simulink model "water_hopper_biped_FCPG_split"  (Simulink 8.0)
settings: Solver=ode23t  StartTime=0.0  StopTime=6  MaxStep=1e-3  RelTol=1e-3
values from neighbouring files (symbols this model uses):
  alpha = 30    [SimParam_FCPG.m]
  Amp = 0.0249    [SimParam_FCPG.m]
  C_d = 0.703    [SimParam_FCPG.m]
  density = 1000    [SimParam_FCPG.m]
  freq = 70    [SimParam_FCPG.m]
  g = 9.81    [SimParam_FCPG.m]
  leg_length = Amp    (= 0.0249)    [SimParam_FCPG.m]
  mass = 0.05    [SimParam_FCPG.m]
  omega_0 = [60 60]'    [SimParam_FCPG.m]
  S1 = (pi*r1^2)*area    (= 0.00115422114093)    [SimParam_FCPG.m]
  S2 = (pi*r2^2)*area    (= 7.21388213081e-05)    [SimParam_FCPG.m]
  tau = 0.001    [SimParam_FCPG.m]
undefined symbols (not defined in the file or in its folder): b, Fratio, k
undefined symbols (not defined in the file): amp, RL_lag, W_coupling, y_0
libraries: mblibv1 x16, dspstat3 x1, simulink x1, dspinverses x1
settings Model: Creator=Metti  LastModifiedBy=nitisht
settings SolverCC: ZeroCrossControl=DisableAll
settings DataIOCC: SignalLoggingSaveFormat=ModelDataLogs
settings DebuggingCC: FcnCallInpInsideContextMsg=EnableAllAsWarning
settings ConfigurationSet: Description=SimMechanics 2G

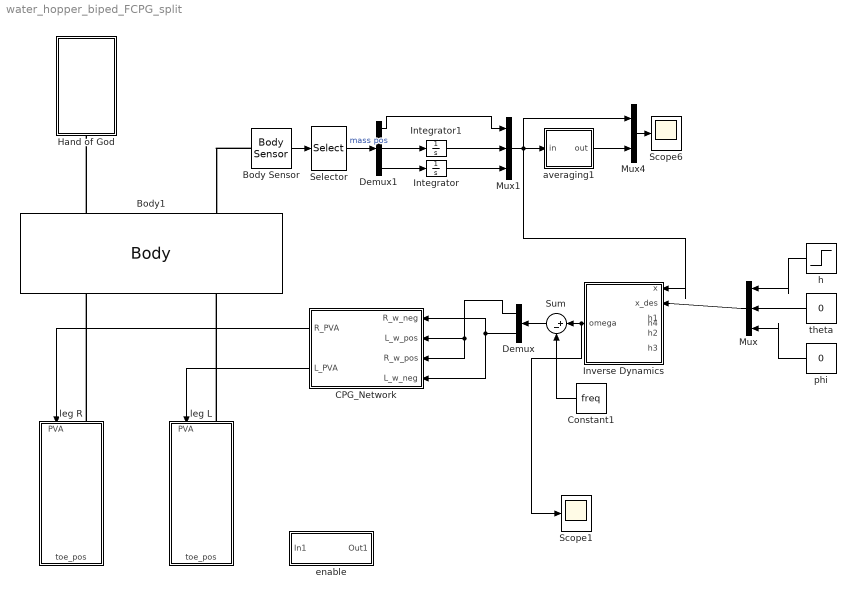
== system water_hopper_biped_FCPG_split ==
  Body Sensor : mblibv1/Sensors &  Actuators/Body Sensor  UpdateFromCAD=off  PhysicalDomain=Mechanical  PortType=blob  Muxed=on  Pose=off  Angle=on  AngleUnits=deg  ArcVelocity=on  ArcVelocityUnits=rad/s  ArcAcceleration=off  ArcAccelerationUnits=deg/s^2  CoordPosition=on  CoordPositionUnits=m  Velocity=off  VelocityUnits=m/s  Acceleration=off  AccelerationUnits=m/s^2  Quaternion=on  QuaternionDT=off  QuaternionDDT=off  QuaternionUnits=off  OutputVector=[1]  ActiveIO=on  Width=3  DialogClass=MechanicalSensorBlock  ReferenceFrame=Absolute (World)
  Body1 : mblibv1/Bodies/Body  LConnTagsString=CS1|CS2  RConnTagsString=CS3|CS4  UpdateFromCAD=off  DialogClass=MechanicalBodyBlock  Mass=mass  MassUnits=kg  InertiaUnits=kg*m^2  Inertia=eye(3)  Shape=Cylinder  ShapeDims=[1 1]  ShapeUnits=m  ShapeUse=false  Density=1  DensityUnits=kg/m^3  DensityUse=false  GraphicsMode=MACHINE_DEFAULT  BodyColorSelMode=MACHINE_DEFAULT  BodyColor=[1 0 0]  AttachedToCS=CG  CG=Left$CG$[0 0 0]$WORLD$WORLD$m$[0 0 0]$Euler X-Y-Z$deg$WORLD$false$none  WorkingFrames=Left$CS1$[0 0 0]$CG$CG$m$[0 0 0]$Euler X-Y-Z$deg$WORLD$true$none#Left$CS2$[0 0 0]$CG$CG$m$[0 0 0]$Euler X-Y-Z$deg$WORLD$true$none#Right$CS3$[0 0 0]$CG$CG$m$[0 0 0]$Euler X-Y-Z$deg$WORLD$true$none#Right$CS4$[0 0 0]$CG$CG$m$[0 0 0]$Euler X-Y-Z$deg$WORLD$true$none  CGPos=[0 0 0]  CGRot=[0 0 0]  CS0Pos=[]  CS0Rot=[]  CS1Pos=[0 0 0]  CS1Rot=[0 0 0]  CS2Pos=[0 0 0]  CS2Rot=[0 0 0]  CS3Pos=[0 0 0]  CS3Rot=[0 0 0]  CS4Pos=[0 0 0]  CS4Rot=[0 0 0]  CS5Pos=[]  CS5Rot=[]  CS6Pos=[]  CS6Rot=[]  CS7Pos=[]  CS7Rot=[]  CS8Pos=[]  CS8Rot=[]  CS9Pos=[]  CS9Rot=[]  CS10Pos=[]  CS10Rot=[]  CS11Pos=[]  CS11Rot=[]  CS12Pos=[]  CS12Rot=[]  CS13Pos=[]  CS13Rot=[]  CS14Pos=[]  CS14Rot=[]  CS15Pos=[]  CS15Rot=[]  CS16Pos=[]  CS16Rot=[]  CS17Pos=[]  CS17Rot=[]  CS18Pos=[]  CS18Rot=[]  CS19Pos=[]  CS19Rot=[]  CS20Pos=[]  CS20Rot=[]
  CPG_Network : Subsystem
  Constant1 : Constant  Value=freq
  Demux : Demux  Outputs=2
  Demux1 : Demux  Outputs=3
  Hand of God : Subsystem
  Integrator : Integrator
  Integrator1 : Integrator
  Inverse Dynamics : Subsystem
  Mux : Mux  Inputs=3
  Mux1 : Mux  Inputs=3
  Mux4 : Mux  Inputs=2
  Scope1 : Scope
      settings: TimeRange=0.00234049245184974  YMin=53.02063772134064  YMax=53.05517753304328  SaveName=omega_control
  Scope6 : Scope
      settings: YMin=0  YMax=0.0175  SaveName=ball_position
  Selector : Selector  InputPortWidth=6  IndexOptions=Index vector (dialog)  Indices=[2 4 5]  OutputSizes=1
  Sum : Sum  Inputs=|+-
  averaging1 : Subsystem  mask{T_win=2*pi/freq*2, x_init=y_0}
      mask prompts: T_win "window (s)"; x_init "Initial condition"
  enable : Subsystem
  h : Step  Time=3  Before=.01  After=.015  SampleTime=0
  leg L : Subsystem
  leg R : Subsystem
  phi : Constant  Value=0
  theta : Constant  Value=0
  wires:
  Body Sensor/1 -> Selector/1
  Mux4/1 -> Scope6/1
  CPG_Network/1(R_PVA) -> leg R/1(PVA)
  CPG_Network/2(L_PVA) -> leg L/1(PVA)
  averaging1/1(out) -> Mux4/2
  Demux/1 -> CPG_Network/3(R_w_pos), CPG_Network/2(L_w_pos)
  Demux/2 -> CPG_Network/4(L_w_neg), CPG_Network/1(R_w_neg)
  Sum/1 -> Demux/1
  Constant1/1 -> Sum/2
  Inverse Dynamics/1(omega) -> Scope1/1, Sum/1
  h/1 -> Mux/1
  theta/1 -> Mux/2
  phi/1 -> Mux/3
  Mux/1 -> Inverse Dynamics/2(x_des)
  Selector/1 -> Demux1/1  "mass pos"
  Demux1/3 -> Integrator/1
  Demux1/2 -> Integrator1/1
  Mux1/1 -> Inverse Dynamics/1(x), Mux4/1, averaging1/1(in)
  Demux1/1 -> Mux1/1
  Integrator1/1 -> Mux1/2
  Integrator/1 -> Mux1/3
  connections:
  Body Sensor/LConn1 -- Body1/LConn2
  leg R/LConn1 -- Body1/RConn1
  Body1/LConn1 -- Hand of God/LConn1
  leg L/LConn1 -- Body1/RConn2

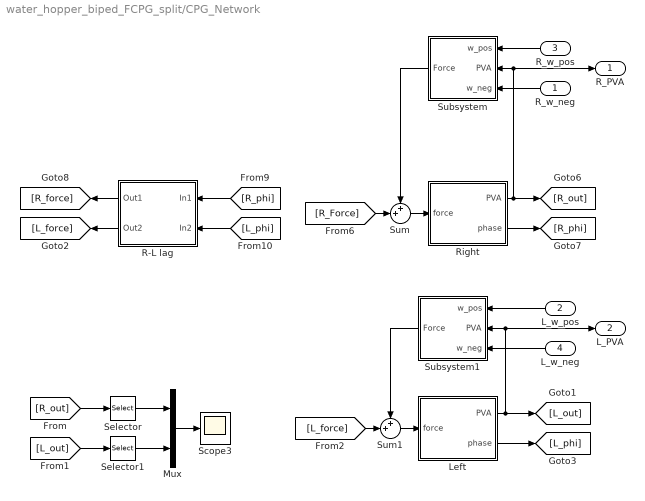
== system water_hopper_biped_FCPG_split/CPG_Network ==
  R_w_neg : Inport
  L_w_pos : Inport  Port=2
  R_w_pos : Inport  Port=3
  L_w_neg : Inport  Port=4
  Left : Subsystem  mask{Amp=amp, Offset=0, init_phi=pi}
      mask prompts: Amp "Amplitude"; init_phi "Initial Phase"
  Mux : Mux  Inputs=2
  R-L lag : Subsystem  mask{d_phase=RL_lag, coupling_weight=W_coupling}
      mask prompts: d_phase "Phase Lag"; coupling_weight "Coupling Weight"
  Right : Subsystem  mask{Amp=amp, Offset=0, init_phi=0}
      mask prompts: Amp "Amplitude"; init_phi "Initial Phase"
  Scope3 : Scope
      settings: TimeRange=3  YMin=-0.025  YMax=0.025  SaveName=Output
  Selector : Selector  InputPortWidth=3  IndexOptions=Index vector (dialog)  Indices=[1]  OutputSizes=1
  Selector1 : Selector  InputPortWidth=3  IndexOptions=Index vector (dialog)  Indices=[1]  OutputSizes=1
  Subsystem : Subsystem
  Subsystem1 : Subsystem
  Sum : Sum  Inputs=++|
  Sum1 : Sum  Inputs=++|
  R_PVA : Outport
  L_PVA : Outport  Port=2
  wires:
  Mux/1 -> Scope3/1
  Left/2(phase) -> [L_phi]
  Right/2(phase) -> [R_phi]
  [L_phi] -> R-L lag/2(In2)
  [R_phi] -> R-L lag/1(In1)
  R-L lag/1(Out1) -> [R_force]
  R-L lag/2(Out2) -> [L_force]
  Right/1(PVA) -> R_PVA/1, Subsystem/2(PVA), [R_out]
  [L_force] -> Sum1/2
  Sum1/1 -> Left/1(force)
  Sum/1 -> Right/1(force)
  [R_Force] -> Sum/2
  [L_out] -> Selector1/1
  Selector1/1 -> Mux/2
  Selector/1 -> Mux/1
  [R_out] -> Selector/1
  R_w_pos/1 -> Subsystem/1(w_pos)
  R_w_neg/1 -> Subsystem/3(w_neg)
  Subsystem/1(Force) -> Sum/1
  L_w_pos/1 -> Subsystem1/1(w_pos)
  L_w_neg/1 -> Subsystem1/3(w_neg)
  Left/1(PVA) -> Subsystem1/2(PVA), L_PVA/1, [L_out]
  Subsystem1/1(Force) -> Sum1/1

== system water_hopper_biped_FCPG_split/Hand of God ==
  Ground : mblibv1/Bodies/Ground  UpdateFromCAD=off  LeftPortType=env  RightPortType=workingframe  PhysicalDomain=Mechanical  DialogClass=GroundBlock  CoordPosition=[0 0 0]  CoordPositionUnits=m  StateVectorMgrId=-1  MachineId=[0 0]  ShowEnvPort=on
  Joint Initial Condition : mblibv1/Sensors &  Actuators/Joint Initial Condition  UpdateFromCAD=off  LeftPortType=blob  RightPortType=blob  PhysicalDomain=mechanical  DialogClass=InitialConditionBlock  InitialConditions=P1$true$y_0$m$deg$0$m/s$deg/s#P2$false$0$m$deg$0$m/s$deg/s#P3$false$0$m$deg$0$m/s$deg/s#R1$false$0$m$deg$0$m/s$deg/s#R2$false$0$m$deg$0$m/s$deg/s#R3$false$0$m$deg$0$m/s$deg/s#S$false$0$m$deg$0$m/s$deg/s  P1PIC=y_0  P1VIC=0  P2PIC=0  P2VIC=0  P3PIC=0  P3VIC=0  R1PIC=0  R1VIC=0  R2PIC=0  R2VIC=0  R3PIC=0  R3VIC=0  SPIC=0  SVIC=0
  Machine Environment : mblibv1/Bodies/Machine Environment  PortType=env  PhysicalDomain=Mechanical  DialogTemplateClass=MECH.MachineEnvironment  SyncWhenCopied=off  Gravity=[0 -g 0]  GravityUnits=m/s^2  GravityAsSignal=off  Dimensionality=Auto-detect  AnalysisType=Forward dynamics  LinearAssemblyTolerance=1e-3  LinearAssemblyToleranceUnits=m  AngularAssemblyTolerance=1e-3  AngularAssemblyToleranceUnits=rad  ConstraintSolverType=Stabilizing  ConstraintRelTolerance=1e-4  ConstraintAbsTolerance=1e-4  UseRobustSingularityHandling=off  RedundancyAnalysisToleranceType=Automatically select tolerance  RedundancyAnalysisTolerance=1e-14  StatePerturbationType=Fixed  PerturbationSize=1e-5  VisualizeMachine=on  BodyVisualizationType=Use model default body geometries  BodyColorSelMode=Use model default  DefaultBodyColor=[1 0 0]
  Prismatic : mblibv1/Joints/Prismatic  LConnTagsString=__newl0|SA1  RConnTagsString=__newr0  UpdateFromCAD=off  NumSAPorts=1  CutJoint=off  MarkAsCut=off  Primitives=prismatic  PrimitiveProps=P1$World$[0 1 0]$prismatic  DialogClass=JointBlock  P1Axis=[0 1 0]
  Conn1 : PMIOPort  Port=1  Side=Left
  connections:
  Conn1/RConn1 -- Prismatic/RConn1
  Machine Environment/RConn1 -- Ground/LConn1
  Ground/RConn1 -- Prismatic/LConn1
  Joint Initial Condition/RConn1 -- Prismatic/LConn2

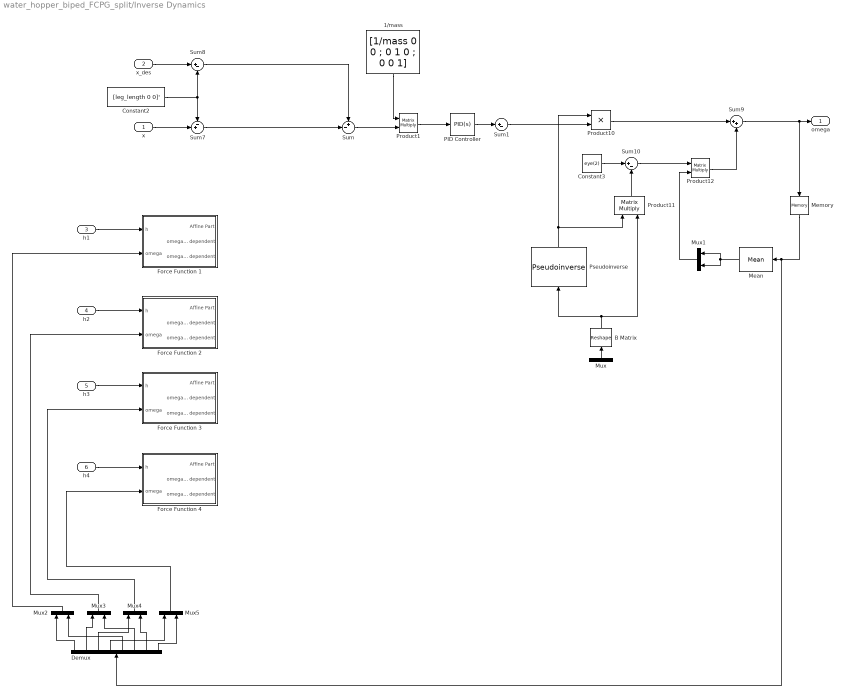
== system water_hopper_biped_FCPG_split/Inverse Dynamics ==
  x : Inport
  x_des : Inport  Port=2
  h1 : Inport  Port=3
  h2 : Inport  Port=4
  h3 : Inport  Port=5
  h4 : Inport  Port=6
  1/mass : Constant  Value=[1/mass 0 0 ; 0 1 0 ; 0 0 1]
  B Matrix : Reshape  OutputDimensionality=Customize  OutputDimensions=[1,2]
  Constant2 : Constant  Value=[leg_length 0 0]'
  Constant3 : Constant  Value=eye(2)
  Demux : Demux  Outputs=8
  Force Function 1 : Subsystem
  Force Function 2 : Subsystem
  Force Function 3 : Subsystem
  Force Function 4 : Subsystem
  Mean : dspstat3/Mean  run=off  reset_popup=None  InputProcessing=Columns as channels (frame based)  directionMode=Entire input  dimension=1  treatSBRowAsCol=on  roiEnable=off  roiType=Rectangles  roiPortion=Entire ROI  roiOutput=Individual statistics for each ROI  roiFlag=off  outputDataTypeStr=Inherit: Same as accumulator  outputLastDataTypeStr=Inherit: Same as accumulator  outputMin=[]  outputMax=[]  roundingMode=Floor  overflowMode=off
  Memory : Memory  X0=omega_0
  Mux{,1..5} (6 alike) : Mux  Inputs=2
  PID Controller : simulink/Continuous/PID Controller  Controller=PID  TimeDomain=Continuous-time  SampleTime=1  IntegratorMethod=Forward Euler  FilterMethod=Forward Euler  Form=Parallel  P=500  I=1000  D=0  N=100  InitialConditionSource=internal  InitialConditionForIntegrator=0  InitialConditionForFilter=0  ExternalReset=none  LimitOutput=off  UpperSaturationLimit=inf  LowerSaturationLimit=-inf  LinearizeAsGain=on  AntiWindupMode=none  Kb=1  TrackingMode=off  Kt=1  PParamMin=[]  PParamMax=[]  IParamMin=[]  IParamMax=[]  DParamMin=[]  DParamMax=[]  NParamMin=[]  NParamMax=[]  KbParamMin=[]  KbParamMax=[]  KtParamMin=[]  KtParamMax=[]  POutMin=[]  POutMax=[]  IOutMin=[]  IOutMax=[]  DOutMin=[]  DOutMax=[]  NOutMin=[]  NOutMax=[]  KbOutMin=[]  KbOutMax=[]  KtOutMin=[]  KtOutMax=[]  IntegratorOutMin=[]  IntegratorOutMax=[]  FilterOutMin=[]  FilterOutMax=[]  SumOutMin=[]  SumOutMax=[]  SumI1OutMin=[]  SumI1OutMax=[]  SumI2OutMin=[]  SumI2OutMax=[]  SumI3OutMin=[]  SumI3OutMax=[]  SumDOutMin=[]  SumDOutMax=[]  SaturationOutMin=[]  SaturationOutMax=[]  IntegratorContinuousStateAttributes=''  IntegratorStateMustResolveToSignalObject=off  IntegratorRTWStateStorageClass=Auto  FilterContinuousStateAttributes=''  FilterStateMustResolveToSignalObject=off  FilterRTWStateStorageClass=Auto
  Product1 : Product  Multiplication=Matrix(*)  RndMeth=Zero
  Product10 : Product  RndMeth=Zero
  Product11 : Product  Multiplication=Matrix(*)  RndMeth=Zero
  Product12 : Product  Multiplication=Matrix(*)  RndMeth=Zero
  Pseudoinverse : dspinverses/Pseudoinverse  wanterr=off
  Sum : Sum  Inputs=+-|
  Sum1 : Sum  Inputs=|+-
  Sum10 : Sum  Inputs=|+-
  Sum7 : Sum  Inputs=-+|
  Sum8 : Sum  Inputs=|+-
  Sum9 : Sum  Inputs=|++
  omega : Outport
  wires:
  Memory/1 -> Demux/1, Mean/1
  PID Controller/1 -> Sum1/1
  Sum/1 -> Product1/2
  Mux/1 -> B Matrix/1
  B Matrix/1 -> Product11/2, Pseudoinverse/1
  Sum7/1 -> Sum/2
  x/1 -> Sum7/2
  Constant2/1 -> Sum7/1, Sum8/2
  x_des/1 -> Sum8/1
  Sum8/1 -> Sum/1
  Pseudoinverse/1 -> Product11/1, Product10/1
  Sum1/1 -> Product10/2
  Product10/1 -> Sum9/1
  Product11/1 -> Sum10/2
  Constant3/1 -> Sum10/1
  Sum10/1 -> Product12/1
  Product12/1 -> Sum9/2
  Sum9/1 -> Memory/1, omega/1
  Mean/1 -> Mux1/2, Mux1/1
  Mux1/1 -> Product12/2
  Product1/1 -> PID Controller/1
  1/mass/1 -> Product1/1
  h4/1 -> Force Function 4/1(h)
  h3/1 -> Force Function 3/1(h)
  h2/1 -> Force Function 2/1(h)
  h1/1 -> Force Function 1/1(h)
  Demux/1 -> Mux2/1
  Demux/5 -> Mux2/2
  Demux/2 -> Mux3/1
  Demux/6 -> Mux3/2
  Demux/3 -> Mux4/1
  Demux/7 -> Mux4/2
  Demux/4 -> Mux5/1
  Demux/8 -> Mux5/2
  Mux2/1 -> Force Function 1/2(omega)
  Mux3/1 -> Force Function 2/2(omega)
  Mux4/1 -> Force Function 3/2(omega)
  Mux5/1 -> Force Function 4/2(omega)

== system water_hopper_biped_FCPG_split/averaging1 ==
  in : Inport
  Constant1 : Constant  Value=x_init
  Gain : Gain  Gain=1/T_win
  Integrator1 : Integrator
  Sum : Sum  Inputs=+-|
  Sum1 : Sum  Inputs=-+|
  Sum3 : Sum  Inputs=++|
  Transport Delay : TransportDelay  DelayTime=T_win
  out : Outport
  wires:
  in/1 -> Sum1/2
  Gain/1 -> Sum3/2
  Constant1/1 -> Sum3/1, Sum1/1
  Sum1/1 -> Integrator1/1
  Transport Delay/1 -> Sum/2
  Integrator1/1 -> Sum/1, Transport Delay/1
  Sum3/1 -> out/1
  Sum/1 -> Gain/1

== system water_hopper_biped_FCPG_split/enable ==
  In1 : Inport
  Constant1 : Constant
  Derivative : Derivative
  Gain : Gain  Gain=.5
  Sign : Signum
  Sum1 : Sum  Inputs=|-+
  Out1 : Outport
  wires:
  Derivative/1 -> Sign/1
  Constant1/1 -> Sum1/2
  Sign/1 -> Sum1/1
  Gain/1 -> Out1/1
  In1/1 -> Derivative/1
  Sum1/1 -> Gain/1

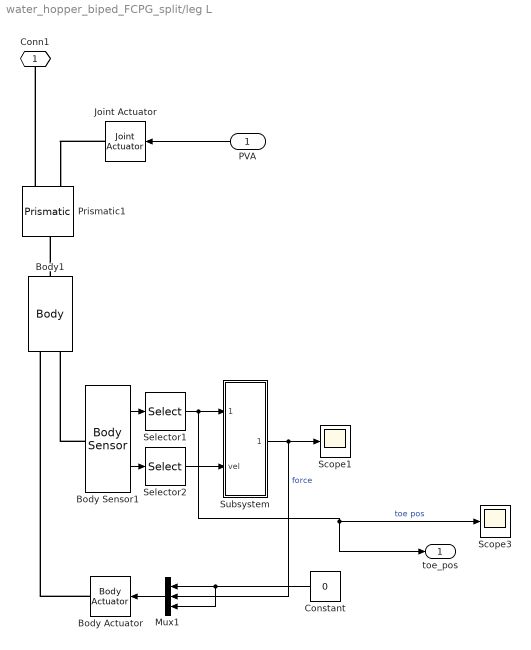
== system water_hopper_biped_FCPG_split/leg L ==
  PVA : Inport
  Body Actuator : mblibv1/Sensors &  Actuators/Body Actuator  UpdateFromCAD=off  PhysicalDomain=Mechanical  PortType=blob  ActuationStyle=Force  AngleUnits=deg  ArcVelocityUnits=deg/s  ArcAccelerationUnits=deg/s^2  CoordPositionUnits=m  VelocityUnits=m/s  AccelerationUnits=m/s^2  ForceUnits=N  TorqueUnits=N-m  ActiveIO=on  Width=3  DialogClass=MechanicalActuatorBlock  ReferenceFrame=Absolute (World)  Angle=off  CoordPosition=on  Force=on  Torque=off
  Body Sensor1 : mblibv1/Sensors &  Actuators/Body Sensor  UpdateFromCAD=off  PhysicalDomain=Mechanical  PortType=blob  Muxed=off  Pose=off  Angle=on  AngleUnits=deg  ArcVelocity=off  ArcVelocityUnits=deg/s  ArcAcceleration=off  ArcAccelerationUnits=deg/s^2  CoordPosition=on  CoordPositionUnits=m  Velocity=on  VelocityUnits=m/s  Acceleration=off  AccelerationUnits=m/s^2  Quaternion=on  QuaternionDT=off  QuaternionDDT=off  QuaternionUnits=off  OutputVector=[1]  ActiveIO=on  Width=6  DialogClass=MechanicalSensorBlock  ReferenceFrame=Absolute (World)
  Body1 : mblibv1/Bodies/Body  LConnTagsString=CS1  RConnTagsString=CS2|CS3  UpdateFromCAD=off  DialogClass=MechanicalBodyBlock  Mass=0  MassUnits=kg  InertiaUnits=kg*m^2  Inertia=zeros(3)  Shape=Cylinder  ShapeDims=[1 1]  ShapeUnits=m  ShapeUse=false  Density=1  DensityUnits=kg/m^3  DensityUse=false  GraphicsMode=MACHINE_DEFAULT  BodyColorSelMode=MACHINE_DEFAULT  BodyColor=[1 0 0]  AttachedToCS=CG  CG=Left$CG$[0 -leg_length 0]$CS1$CS1$m$[0 0 0]$Euler X-Y-Z$deg$WORLD$false$none  WorkingFrames=Left$CS1$[0 0 0]$Adjoining$Adjoining$m$[0 0 0]$Euler X-Y-Z$deg$WORLD$true$none#Right$CS2$[0 -leg_length 0]$CS1$CS1$m$[0 0 0]$Euler X-Y-Z$deg$WORLD$true$none#Right$CS3$[0 -leg_length 0]$CS1$CS1$m$[0 0 0]$Euler X-Y-Z$deg$WORLD$true$none  CGPos=[0 -leg_length 0]  CGRot=[0 0 0]  CS0Pos=[]  CS0Rot=[]  CS1Pos=[0 0 0]  CS1Rot=[0 0 0]  CS2Pos=[0 -leg_length 0]  CS2Rot=[0 0 0]  CS3Pos=[0 -leg_length 0]  CS3Rot=[0 0 0]  CS4Pos=[]  CS4Rot=[]  CS5Pos=[]  CS5Rot=[]  CS6Pos=[]  CS6Rot=[]  CS7Pos=[]  CS7Rot=[]  CS8Pos=[]  CS8Rot=[]  CS9Pos=[]  CS9Rot=[]  CS10Pos=[]  CS10Rot=[]  CS11Pos=[]  CS11Rot=[]  CS12Pos=[]  CS12Rot=[]  CS13Pos=[]  CS13Rot=[]  CS14Pos=[]  CS14Rot=[]  CS15Pos=[]  CS15Rot=[]  CS16Pos=[]  CS16Rot=[]  CS17Pos=[]  CS17Rot=[]  CS18Pos=[]  CS18Rot=[]  CS19Pos=[]  CS19Rot=[]  CS20Pos=[]  CS20Rot=[]
  Constant : Constant  Value=0
  Joint Actuator : mblibv1/Sensors &  Actuators/Joint Actuator  UpdateFromCAD=off  PhysicalDomain=Mechanical  PortType=blob  ActuationStyle=Motion  AngleUnits=deg  ArcVelocityUnits=deg/s  ArcAccelerationUnits=deg/s^2  CoordPositionUnits=m  VelocityUnits=m/s  AccelerationUnits=m/s^2  ForceUnits=N  TorqueUnits=N*m  ActiveIO=on  Width=3  DialogClass=MechanicalActuatorBlock  Primitive=P1  ReferenceFrame=Absolute (World)
  Mux1 : Mux  Inputs=3
  Prismatic1 : mblibv1/Joints/Prismatic  LConnTagsString=__newl0|SA1  RConnTagsString=__newr0  UpdateFromCAD=off  NumSAPorts=1  CutJoint=off  MarkAsCut=off  Primitives=prismatic  PrimitiveProps=P1$World$[0 1 0]$prismatic  DialogClass=JointBlock  P1Axis=[0 1 0]
  Scope1 : Scope
      settings: SaveName=force_L
  Scope3 : Scope
      settings: SaveName=toe_position_L
  Selector1 : Selector  InputPortWidth=3  IndexOptions=Index vector (dialog)  Indices=[2]  OutputSizes=1
  Selector2 : Selector  InputPortWidth=3  IndexOptions=Index vector (dialog)  Indices=[2]  OutputSizes=1
  Subsystem : Subsystem
  Conn1 : PMIOPort  Port=1  Side=Left
  toe_pos : Outport
  wires:
  PVA/1 -> Joint Actuator/1
  Constant/1 -> Mux1/3, Mux1/1
  Mux1/1 -> Body Actuator/1
  Subsystem/1(force) -> Mux1/2, Scope1/1  "force"
  Selector2/1 -> Subsystem/2(vel)
  Selector1/1 -> toe_pos/1, Scope3/1, Subsystem/1(pos)  "toe pos"
  Body Sensor1/2 -> Selector2/1
  Body Sensor1/1 -> Selector1/1
  connections:
  Joint Actuator/RConn1 -- Prismatic1/LConn2
  Prismatic1/LConn1 -- Conn1/RConn1
  Body Sensor1/LConn1 -- Body1/RConn2
  Body Actuator/RConn1 -- Body1/RConn1
  Body1/LConn1 -- Prismatic1/RConn1

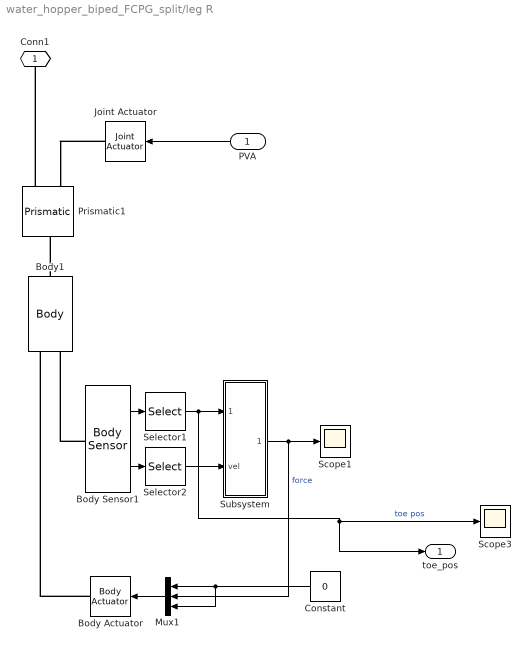
== system water_hopper_biped_FCPG_split/leg R ==
  PVA : Inport
  Body Actuator : mblibv1/Sensors &  Actuators/Body Actuator  UpdateFromCAD=off  PhysicalDomain=Mechanical  PortType=blob  ActuationStyle=Force  AngleUnits=deg  ArcVelocityUnits=deg/s  ArcAccelerationUnits=deg/s^2  CoordPositionUnits=m  VelocityUnits=m/s  AccelerationUnits=m/s^2  ForceUnits=N  TorqueUnits=N-m  ActiveIO=on  Width=3  DialogClass=MechanicalActuatorBlock  ReferenceFrame=Absolute (World)  Angle=off  CoordPosition=on  Force=on  Torque=off
  Body Sensor1 : mblibv1/Sensors &  Actuators/Body Sensor  UpdateFromCAD=off  PhysicalDomain=Mechanical  PortType=blob  Muxed=off  Pose=off  Angle=on  AngleUnits=deg  ArcVelocity=off  ArcVelocityUnits=deg/s  ArcAcceleration=off  ArcAccelerationUnits=deg/s^2  CoordPosition=on  CoordPositionUnits=m  Velocity=on  VelocityUnits=m/s  Acceleration=off  AccelerationUnits=m/s^2  Quaternion=on  QuaternionDT=off  QuaternionDDT=off  QuaternionUnits=off  OutputVector=[1]  ActiveIO=on  Width=6  DialogClass=MechanicalSensorBlock  ReferenceFrame=Absolute (World)
  Body1 : mblibv1/Bodies/Body  LConnTagsString=CS1  RConnTagsString=CS2|CS3  UpdateFromCAD=off  DialogClass=MechanicalBodyBlock  Mass=0  MassUnits=kg  InertiaUnits=kg*m^2  Inertia=zeros(3)  Shape=Cylinder  ShapeDims=[1 1]  ShapeUnits=m  ShapeUse=false  Density=1  DensityUnits=kg/m^3  DensityUse=false  GraphicsMode=MACHINE_DEFAULT  BodyColorSelMode=MACHINE_DEFAULT  BodyColor=[1 0 0]  AttachedToCS=CG  CG=Left$CG$[0 -leg_length 0]$CS1$CS1$m$[0 0 0]$Euler X-Y-Z$deg$WORLD$false$none  WorkingFrames=Left$CS1$[0 0 0]$Adjoining$Adjoining$m$[0 0 0]$Euler X-Y-Z$deg$WORLD$true$none#Right$CS2$[0 -leg_length 0]$CS1$CS1$m$[0 0 0]$Euler X-Y-Z$deg$WORLD$true$none#Right$CS3$[0 -leg_length 0]$CS1$CS1$m$[0 0 0]$Euler X-Y-Z$deg$WORLD$true$none  CGPos=[0 -leg_length 0]  CGRot=[0 0 0]  CS0Pos=[]  CS0Rot=[]  CS1Pos=[0 0 0]  CS1Rot=[0 0 0]  CS2Pos=[0 -leg_length 0]  CS2Rot=[0 0 0]  CS3Pos=[0 -leg_length 0]  CS3Rot=[0 0 0]  CS4Pos=[]  CS4Rot=[]  CS5Pos=[]  CS5Rot=[]  CS6Pos=[]  CS6Rot=[]  CS7Pos=[]  CS7Rot=[]  CS8Pos=[]  CS8Rot=[]  CS9Pos=[]  CS9Rot=[]  CS10Pos=[]  CS10Rot=[]  CS11Pos=[]  CS11Rot=[]  CS12Pos=[]  CS12Rot=[]  CS13Pos=[]  CS13Rot=[]  CS14Pos=[]  CS14Rot=[]  CS15Pos=[]  CS15Rot=[]  CS16Pos=[]  CS16Rot=[]  CS17Pos=[]  CS17Rot=[]  CS18Pos=[]  CS18Rot=[]  CS19Pos=[]  CS19Rot=[]  CS20Pos=[]  CS20Rot=[]
  Constant : Constant  Value=0
  Joint Actuator : mblibv1/Sensors &  Actuators/Joint Actuator  UpdateFromCAD=off  PhysicalDomain=Mechanical  PortType=blob  ActuationStyle=Motion  AngleUnits=deg  ArcVelocityUnits=deg/s  ArcAccelerationUnits=deg/s^2  CoordPositionUnits=m  VelocityUnits=m/s  AccelerationUnits=m/s^2  ForceUnits=N  TorqueUnits=N*m  ActiveIO=on  Width=3  DialogClass=MechanicalActuatorBlock  Primitive=P1  ReferenceFrame=Absolute (World)
  Mux1 : Mux  Inputs=3
  Prismatic1 : mblibv1/Joints/Prismatic  LConnTagsString=__newl0|SA1  RConnTagsString=__newr0  UpdateFromCAD=off  NumSAPorts=1  CutJoint=off  MarkAsCut=off  Primitives=prismatic  PrimitiveProps=P1$World$[0 1 0]$prismatic  DialogClass=JointBlock  P1Axis=[0 1 0]
  Scope1 : Scope
      settings: SaveName=force_L
  Scope3 : Scope
      settings: SaveName=toe_position_L
  Selector1 : Selector  InputPortWidth=3  IndexOptions=Index vector (dialog)  Indices=[2]  OutputSizes=1
  Selector2 : Selector  InputPortWidth=3  IndexOptions=Index vector (dialog)  Indices=[2]  OutputSizes=1
  Subsystem : Subsystem
  Conn1 : PMIOPort  Port=1  Side=Left
  toe_pos : Outport
  wires:
  Body Sensor1/1 -> Selector1/1
  Body Sensor1/2 -> Selector2/1
  Selector1/1 -> Subsystem/1(pos), Scope3/1, toe_pos/1  "toe pos"
  Selector2/1 -> Subsystem/2(vel)
  Subsystem/1(force) -> Scope1/1, Mux1/2  "force"
  Mux1/1 -> Body Actuator/1
  Constant/1 -> Mux1/1, Mux1/3
  PVA/1 -> Joint Actuator/1
  connections:
  Body1/LConn1 -- Prismatic1/RConn1
  Body Actuator/RConn1 -- Body1/RConn1
  Body Sensor1/LConn1 -- Body1/RConn2
  Prismatic1/LConn1 -- Conn1/RConn1
  Joint Actuator/RConn1 -- Prismatic1/LConn2

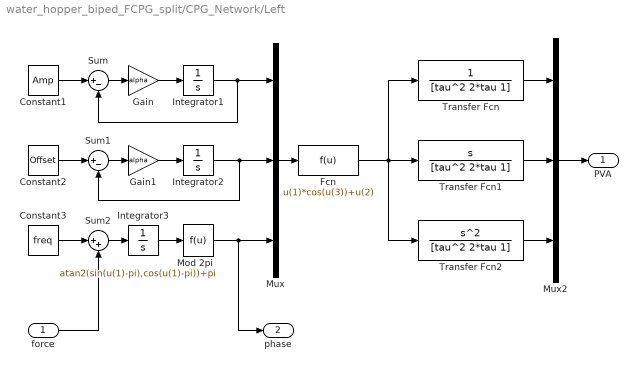
== system water_hopper_biped_FCPG_split/CPG_Network/Left ==
  force : Inport
  Constant1 : Constant  Value=Amp
  Constant2 : Constant  Value=Offset
  Constant3 : Constant  Value=freq
  Fcn : Fcn  Expr=u(1)*cos(u(3))+u(2)
  Gain : Gain  Gain=alpha
  Gain1 : Gain  Gain=alpha
  Integrator1 : Integrator
  Integrator2 : Integrator
  Integrator3 : Integrator  InitialCondition=init_phi + 0.01*rand
  Mod 2pi : Fcn  Expr=atan2(sin(u(1)-pi),cos(u(1)-pi))+pi
  Mux : Mux  Inputs=3
  Mux2 : Mux  Inputs=3
  Sum : Sum  Inputs=|+-
  Sum1 : Sum  Inputs=|+-
  Sum2 : Sum  Inputs=|++
  Transfer Fcn : TransferFcn  Denominator=[tau^2 2*tau 1]
  Transfer Fcn1 : TransferFcn  Numerator=[1 0]  Denominator=[tau^2 2*tau 1]
  Transfer Fcn2 : TransferFcn  Numerator=[1 0 0]  Denominator=[tau^2 2*tau 1]
  PVA : Outport
  phase : Outport  Port=2
  wires:
  Mux2/1 -> PVA/1
  Fcn/1 -> Transfer Fcn1/1, Transfer Fcn/1, Transfer Fcn2/1
  Transfer Fcn1/1 -> Mux2/2
  Transfer Fcn/1 -> Mux2/1
  Transfer Fcn2/1 -> Mux2/3
  force/1 -> Sum2/2
  Sum2/1 -> Integrator3/1
  Constant3/1 -> Sum2/1
  Integrator3/1 -> Mod 2pi/1
  Mod 2pi/1 -> Mux/3, phase/1
  Mux/1 -> Fcn/1
  Gain1/1 -> Integrator2/1
  Constant2/1 -> Sum1/1
  Integrator2/1 -> Mux/2, Sum1/2
  Sum1/1 -> Gain1/1
  Gain/1 -> Integrator1/1
  Constant1/1 -> Sum/1
  Integrator1/1 -> Mux/1, Sum/2
  Sum/1 -> Gain/1

== system water_hopper_biped_FCPG_split/CPG_Network/R-L lag ==
  In1 : Inport
  In2 : Inport  Port=2
  Constant : Constant  Value=d_phase
  Gain : Gain  Gain=-1
  Sum : Sum  Inputs=--+
  sin : Fcn  Expr=coupling_weight*sin(u(1))
  Out1 : Outport
  Out2 : Outport  Port=2
  wires:
  Sum/1 -> sin/1
  sin/1 -> Gain/1, Out1/1
  Constant/1 -> Sum/2
  In1/1 -> Sum/1
  In2/1 -> Sum/3
  Gain/1 -> Out2/1

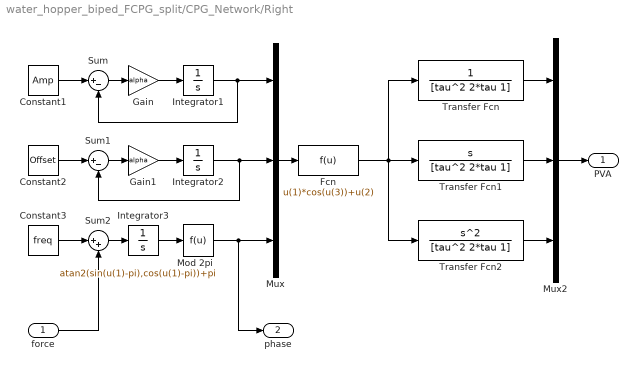
== system water_hopper_biped_FCPG_split/CPG_Network/Right ==
  force : Inport
  Constant1 : Constant  Value=Amp
  Constant2 : Constant  Value=Offset
  Constant3 : Constant  Value=freq
  Fcn : Fcn  Expr=u(1)*cos(u(3))+u(2)
  Gain : Gain  Gain=alpha
  Gain1 : Gain  Gain=alpha
  Integrator1 : Integrator
  Integrator2 : Integrator
  Integrator3 : Integrator  InitialCondition=init_phi + 0.01*rand
  Mod 2pi : Fcn  Expr=atan2(sin(u(1)-pi),cos(u(1)-pi))+pi
  Mux : Mux  Inputs=3
  Mux2 : Mux  Inputs=3
  Sum : Sum  Inputs=|+-
  Sum1 : Sum  Inputs=|+-
  Sum2 : Sum  Inputs=|++
  Transfer Fcn : TransferFcn  Denominator=[tau^2 2*tau 1]
  Transfer Fcn1 : TransferFcn  Numerator=[1 0]  Denominator=[tau^2 2*tau 1]
  Transfer Fcn2 : TransferFcn  Numerator=[1 0 0]  Denominator=[tau^2 2*tau 1]
  PVA : Outport
  phase : Outport  Port=2
  wires:
  Sum/1 -> Gain/1
  Integrator1/1 -> Sum/2, Mux/1
  Constant1/1 -> Sum/1
  Gain/1 -> Integrator1/1
  Sum1/1 -> Gain1/1
  Integrator2/1 -> Sum1/2, Mux/2
  Constant2/1 -> Sum1/1
  Gain1/1 -> Integrator2/1
  Mux/1 -> Fcn/1
  Mod 2pi/1 -> phase/1, Mux/3
  Integrator3/1 -> Mod 2pi/1
  Constant3/1 -> Sum2/1
  Sum2/1 -> Integrator3/1
  force/1 -> Sum2/2
  Transfer Fcn2/1 -> Mux2/3
  Transfer Fcn/1 -> Mux2/1
  Transfer Fcn1/1 -> Mux2/2
  Fcn/1 -> Transfer Fcn2/1, Transfer Fcn/1, Transfer Fcn1/1
  Mux2/1 -> PVA/1

== system water_hopper_biped_FCPG_split/CPG_Network/Subsystem ==
  w_pos : Inport
  PVA : Inport  Port=2
  w_neg : Inport  Port=3
  Product : Product  RndMeth=Zero
  Product1 : Product  RndMeth=Zero
  Sum2 : Sum  Inputs=|++
  enable : Subsystem
  sel : Selector  InputPortWidth=3  IndexOptions=Index vector (dialog)  Indices=[2]  OutputSizes=1
  Force : Outport
  wires:
  Product/1 -> Sum2/1
  w_pos/1 -> Product/1
  w_neg/1 -> Product1/1
  Product1/1 -> Sum2/2
  PVA/1 -> sel/1
  enable/1(pos) -> Product/2
  enable/2(neg) -> Product1/2
  Sum2/1 -> Force/1
  sel/1 -> enable/1(in)

== system water_hopper_biped_FCPG_split/CPG_Network/Subsystem1 ==
  w_pos : Inport
  PVA : Inport  Port=2
  w_neg : Inport  Port=3
  Product : Product  RndMeth=Zero
  Product1 : Product  RndMeth=Zero
  Sum2 : Sum  Inputs=|++
  enable : Subsystem
  sel : Selector  InputPortWidth=3  IndexOptions=Index vector (dialog)  Indices=[2]  OutputSizes=1
  Force : Outport
  wires:
  Product/1 -> Sum2/1
  w_pos/1 -> Product/1
  w_neg/1 -> Product1/1
  Product1/1 -> Sum2/2
  PVA/1 -> sel/1
  enable/1(pos) -> Product/2
  enable/2(neg) -> Product1/2
  Sum2/1 -> Force/1
  sel/1 -> enable/1(in)

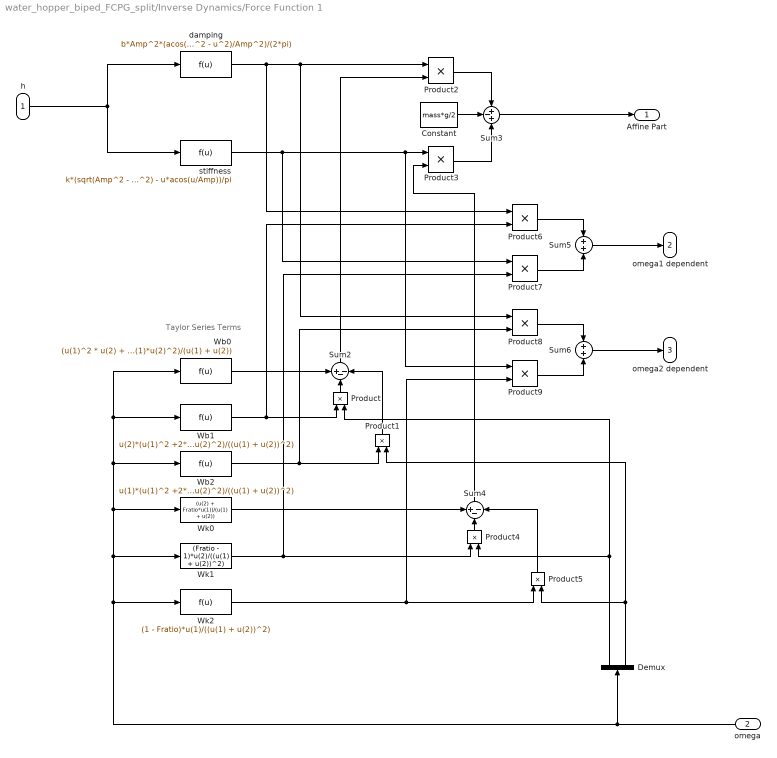
== system water_hopper_biped_FCPG_split/Inverse Dynamics/Force Function 1 ==
  note: Taylor Series Terms
  h : Inport
  omega : Inport  Port=2
  Constant : Constant  Value=mass*g/2
  Demux : Demux  Outputs=2
  Product{,1..9} (10 alike) : Product  RndMeth=Zero
  Sum2 : Sum  Inputs=+--
  Sum3 : Sum  Inputs=+-+
  Sum4 : Sum  Inputs=+--
  Sum5 : Sum  Inputs=+|+
  Sum6 : Sum  Inputs=+|+
  Wb0 : Fcn  Expr=(u(1)^2 * u(2) + Fratio*u(1)*u(2)^2)/(u(1) + u(2))
  Wb1 : Fcn  Expr=u(2)*(u(1)^2 +2*u(1)*u(2) + Fratio*u(2)^2)/((u(1) + u(2))^2)
  Wb2 : Fcn  Expr=u(1)*(u(1)^2 +2*Fratio*u(1)*u(2) + Fratio*u(2)^2)/((u(1) + u(2))^2)
  Wk0 : Fcn  Expr=(u(2) + Fratio*u(1))/(u(1) + u(2))
  Wk1 : Fcn  Expr=(Fratio - 1)*u(2)/((u(1) + u(2))^2)
  Wk2 : Fcn  Expr=(1 - Fratio)*u(1)/((u(1) + u(2))^2)
  damping : Fcn  Expr=b*Amp^2*(acos(u/Amp) - u*sqrt(Amp^2 - u^2)/Amp^2)/(2*pi)
  stiffness : Fcn  Expr=k*(sqrt(Amp^2 - u^2) - u*acos(u/Amp))/pi
  Affine Part : Outport
  omega1 dependent : Outport  Port=2
  omega2 dependent : Outport  Port=3
  wires:
  Product2/1 -> Sum3/1
  Product9/1 -> Sum6/2
  Wb1/1 -> Product6/2, Product/1
  Product4/1 -> Sum4/2
  Wb0/1 -> Sum2/1
  Product7/1 -> Sum5/2
  Wk1/1 -> Product7/2, Product4/1
  Wk0/1 -> Sum4/1
  Product6/1 -> Sum5/1
  Wb2/1 -> Product8/2, Product1/1
  Product/1 -> Sum2/2
  Sum3/1 -> Affine Part/1
  Product1/1 -> Sum2/3
  stiffness/1 -> Product7/1, Product9/1, Product3/1
  Wk2/1 -> Product5/1, Product9/2
  damping/1 -> Product6/1, Product8/1, Product2/1
  Constant/1 -> Sum3/2
  Product5/1 -> Sum4/3
  Product3/1 -> Sum3/3
  Sum5/1 -> omega1 dependent/1
  Sum4/1 -> Product3/2
  omega/1 -> Wb0/1, Wb1/1, Wb2/1, Wk0/1, Wk1/1, Wk2/1, Demux/1
  Sum2/1 -> Product2/2
  Product8/1 -> Sum6/1
  Sum6/1 -> omega2 dependent/1
  Demux/1 -> Product4/2, Product/2
  Demux/2 -> Product5/2, Product1/2
  h/1 -> stiffness/1, damping/1

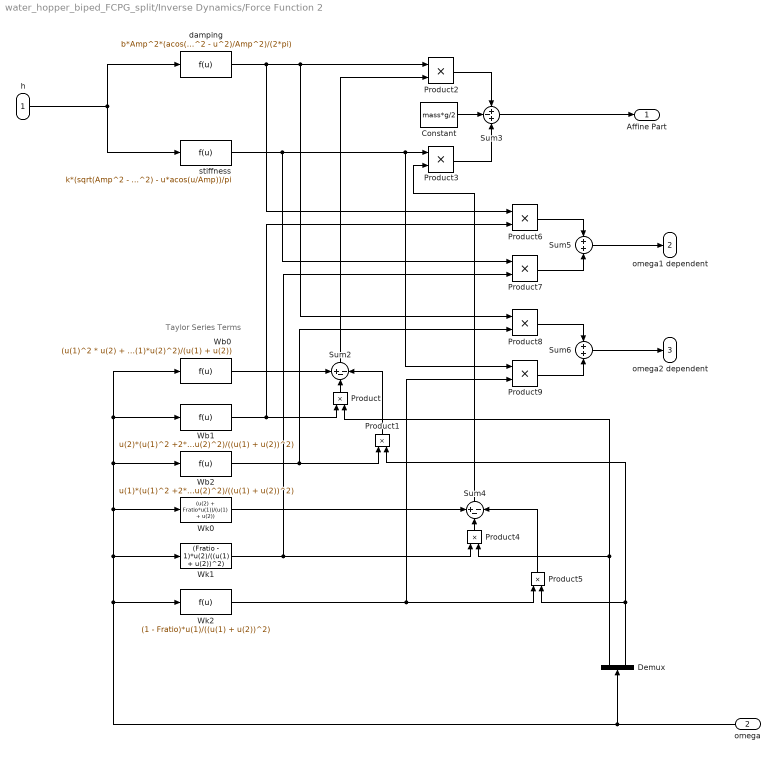
== system water_hopper_biped_FCPG_split/Inverse Dynamics/Force Function 2 ==
  note: Taylor Series Terms
  h : Inport
  omega : Inport  Port=2
  Constant : Constant  Value=mass*g/2
  Demux : Demux  Outputs=2
  Product{,1..9} (10 alike) : Product  RndMeth=Zero
  Sum2 : Sum  Inputs=+--
  Sum3 : Sum  Inputs=+-+
  Sum4 : Sum  Inputs=+--
  Sum5 : Sum  Inputs=+|+
  Sum6 : Sum  Inputs=+|+
  Wb0 : Fcn  Expr=(u(1)^2 * u(2) + Fratio*u(1)*u(2)^2)/(u(1) + u(2))
  Wb1 : Fcn  Expr=u(2)*(u(1)^2 +2*u(1)*u(2) + Fratio*u(2)^2)/((u(1) + u(2))^2)
  Wb2 : Fcn  Expr=u(1)*(u(1)^2 +2*Fratio*u(1)*u(2) + Fratio*u(2)^2)/((u(1) + u(2))^2)
  Wk0 : Fcn  Expr=(u(2) + Fratio*u(1))/(u(1) + u(2))
  Wk1 : Fcn  Expr=(Fratio - 1)*u(2)/((u(1) + u(2))^2)
  Wk2 : Fcn  Expr=(1 - Fratio)*u(1)/((u(1) + u(2))^2)
  damping : Fcn  Expr=b*Amp^2*(acos(u/Amp) - u*sqrt(Amp^2 - u^2)/Amp^2)/(2*pi)
  stiffness : Fcn  Expr=k*(sqrt(Amp^2 - u^2) - u*acos(u/Amp))/pi
  Affine Part : Outport
  omega1 dependent : Outport  Port=2
  omega2 dependent : Outport  Port=3
  wires:
  Product2/1 -> Sum3/1
  Product9/1 -> Sum6/2
  Wb1/1 -> Product6/2, Product/1
  Product4/1 -> Sum4/2
  Wb0/1 -> Sum2/1
  Product7/1 -> Sum5/2
  Wk1/1 -> Product7/2, Product4/1
  Wk0/1 -> Sum4/1
  Product6/1 -> Sum5/1
  Wb2/1 -> Product8/2, Product1/1
  Product/1 -> Sum2/2
  Sum3/1 -> Affine Part/1
  Product1/1 -> Sum2/3
  stiffness/1 -> Product7/1, Product9/1, Product3/1
  Wk2/1 -> Product5/1, Product9/2
  damping/1 -> Product6/1, Product8/1, Product2/1
  Constant/1 -> Sum3/2
  Product5/1 -> Sum4/3
  Product3/1 -> Sum3/3
  Sum5/1 -> omega1 dependent/1
  Sum4/1 -> Product3/2
  omega/1 -> Wb0/1, Wb1/1, Wb2/1, Wk0/1, Wk1/1, Wk2/1, Demux/1
  Sum2/1 -> Product2/2
  Product8/1 -> Sum6/1
  Sum6/1 -> omega2 dependent/1
  Demux/1 -> Product4/2, Product/2
  Demux/2 -> Product5/2, Product1/2
  h/1 -> stiffness/1, damping/1

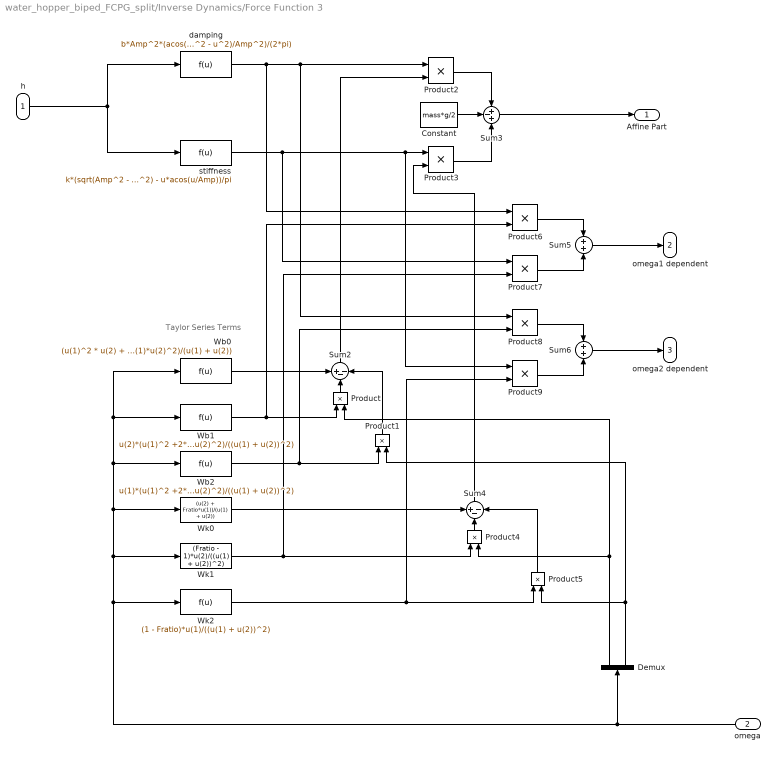
== system water_hopper_biped_FCPG_split/Inverse Dynamics/Force Function 3 ==
  note: Taylor Series Terms
  h : Inport
  omega : Inport  Port=2
  Constant : Constant  Value=mass*g/2
  Demux : Demux  Outputs=2
  Product{,1..9} (10 alike) : Product  RndMeth=Zero
  Sum2 : Sum  Inputs=+--
  Sum3 : Sum  Inputs=+-+
  Sum4 : Sum  Inputs=+--
  Sum5 : Sum  Inputs=+|+
  Sum6 : Sum  Inputs=+|+
  Wb0 : Fcn  Expr=(u(1)^2 * u(2) + Fratio*u(1)*u(2)^2)/(u(1) + u(2))
  Wb1 : Fcn  Expr=u(2)*(u(1)^2 +2*u(1)*u(2) + Fratio*u(2)^2)/((u(1) + u(2))^2)
  Wb2 : Fcn  Expr=u(1)*(u(1)^2 +2*Fratio*u(1)*u(2) + Fratio*u(2)^2)/((u(1) + u(2))^2)
  Wk0 : Fcn  Expr=(u(2) + Fratio*u(1))/(u(1) + u(2))
  Wk1 : Fcn  Expr=(Fratio - 1)*u(2)/((u(1) + u(2))^2)
  Wk2 : Fcn  Expr=(1 - Fratio)*u(1)/((u(1) + u(2))^2)
  damping : Fcn  Expr=b*Amp^2*(acos(u/Amp) - u*sqrt(Amp^2 - u^2)/Amp^2)/(2*pi)
  stiffness : Fcn  Expr=k*(sqrt(Amp^2 - u^2) - u*acos(u/Amp))/pi
  Affine Part : Outport
  omega1 dependent : Outport  Port=2
  omega2 dependent : Outport  Port=3
  wires:
  Product2/1 -> Sum3/1
  Product9/1 -> Sum6/2
  Wb1/1 -> Product6/2, Product/1
  Product4/1 -> Sum4/2
  Wb0/1 -> Sum2/1
  Product7/1 -> Sum5/2
  Wk1/1 -> Product7/2, Product4/1
  Wk0/1 -> Sum4/1
  Product6/1 -> Sum5/1
  Wb2/1 -> Product8/2, Product1/1
  Product/1 -> Sum2/2
  Sum3/1 -> Affine Part/1
  Product1/1 -> Sum2/3
  stiffness/1 -> Product7/1, Product9/1, Product3/1
  Wk2/1 -> Product5/1, Product9/2
  damping/1 -> Product6/1, Product8/1, Product2/1
  Constant/1 -> Sum3/2
  Product5/1 -> Sum4/3
  Product3/1 -> Sum3/3
  Sum5/1 -> omega1 dependent/1
  Sum4/1 -> Product3/2
  omega/1 -> Wb0/1, Wb1/1, Wb2/1, Wk0/1, Wk1/1, Wk2/1, Demux/1
  Sum2/1 -> Product2/2
  Product8/1 -> Sum6/1
  Sum6/1 -> omega2 dependent/1
  Demux/1 -> Product4/2, Product/2
  Demux/2 -> Product5/2, Product1/2
  h/1 -> stiffness/1, damping/1

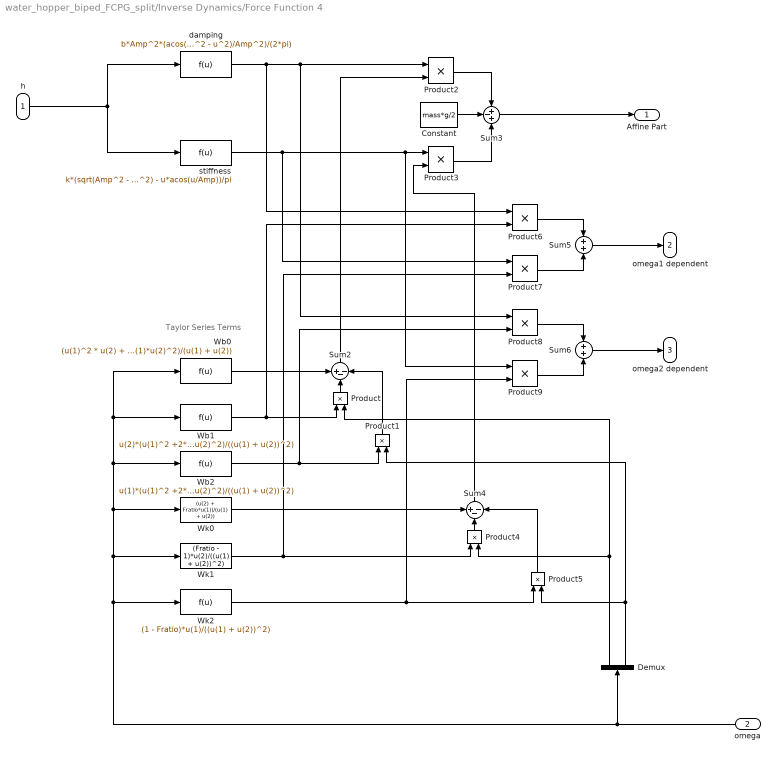
== system water_hopper_biped_FCPG_split/Inverse Dynamics/Force Function 4 ==
  note: Taylor Series Terms
  h : Inport
  omega : Inport  Port=2
  Constant : Constant  Value=mass*g/2
  Demux : Demux  Outputs=2
  Product{,1..9} (10 alike) : Product  RndMeth=Zero
  Sum2 : Sum  Inputs=+--
  Sum3 : Sum  Inputs=+-+
  Sum4 : Sum  Inputs=+--
  Sum5 : Sum  Inputs=+|+
  Sum6 : Sum  Inputs=+|+
  Wb0 : Fcn  Expr=(u(1)^2 * u(2) + Fratio*u(1)*u(2)^2)/(u(1) + u(2))
  Wb1 : Fcn  Expr=u(2)*(u(1)^2 +2*u(1)*u(2) + Fratio*u(2)^2)/((u(1) + u(2))^2)
  Wb2 : Fcn  Expr=u(1)*(u(1)^2 +2*Fratio*u(1)*u(2) + Fratio*u(2)^2)/((u(1) + u(2))^2)
  Wk0 : Fcn  Expr=(u(2) + Fratio*u(1))/(u(1) + u(2))
  Wk1 : Fcn  Expr=(Fratio - 1)*u(2)/((u(1) + u(2))^2)
  Wk2 : Fcn  Expr=(1 - Fratio)*u(1)/((u(1) + u(2))^2)
  damping : Fcn  Expr=b*Amp^2*(acos(u/Amp) - u*sqrt(Amp^2 - u^2)/Amp^2)/(2*pi)
  stiffness : Fcn  Expr=k*(sqrt(Amp^2 - u^2) - u*acos(u/Amp))/pi
  Affine Part : Outport
  omega1 dependent : Outport  Port=2
  omega2 dependent : Outport  Port=3
  wires:
  Product2/1 -> Sum3/1
  Product9/1 -> Sum6/2
  Wb1/1 -> Product6/2, Product/1
  Product4/1 -> Sum4/2
  Wb0/1 -> Sum2/1
  Product7/1 -> Sum5/2
  Wk1/1 -> Product7/2, Product4/1
  Wk0/1 -> Sum4/1
  Product6/1 -> Sum5/1
  Wb2/1 -> Product8/2, Product1/1
  Product/1 -> Sum2/2
  Sum3/1 -> Affine Part/1
  Product1/1 -> Sum2/3
  stiffness/1 -> Product7/1, Product9/1, Product3/1
  Wk2/1 -> Product5/1, Product9/2
  damping/1 -> Product6/1, Product8/1, Product2/1
  Constant/1 -> Sum3/2
  Product5/1 -> Sum4/3
  Product3/1 -> Sum3/3
  Sum5/1 -> omega1 dependent/1
  Sum4/1 -> Product3/2
  omega/1 -> Wb0/1, Wb1/1, Wb2/1, Wk0/1, Wk1/1, Wk2/1, Demux/1
  Sum2/1 -> Product2/2
  Product8/1 -> Sum6/1
  Sum6/1 -> omega2 dependent/1
  Demux/1 -> Product4/2, Product/2
  Demux/2 -> Product5/2, Product1/2
  h/1 -> stiffness/1, damping/1

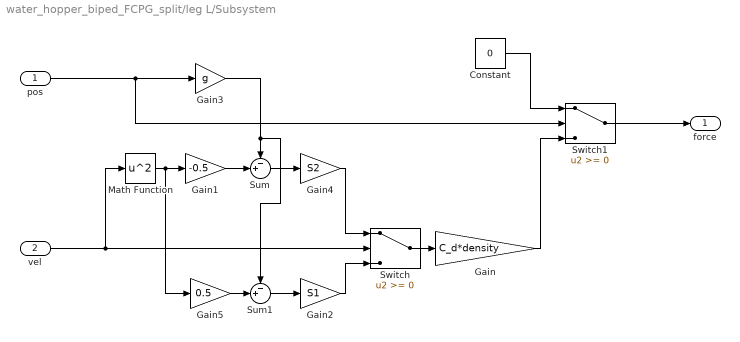
== system water_hopper_biped_FCPG_split/leg L/Subsystem ==
  pos : Inport
  vel : Inport  Port=2
  Constant : Constant  Value=0
  Gain : Gain  Gain=C_d*density
  Gain1 : Gain  Gain=-0.5
  Gain2 : Gain  Gain=S1
  Gain3 : Gain  Gain=g
  Gain4 : Gain  Gain=S2
  Gain5 : Gain  Gain=0.5
  Math Function : Math  Operator=square  SaturateOnIntegerOverflow=on
  Sum : Sum  Inputs=-+|
  Sum1 : Sum  Inputs=-+|
  Switch : Switch  ZeroCross=off
  Switch1 : Switch
  force : Outport
  wires:
  Gain5/1 -> Sum1/2
  Sum1/1 -> Gain2/1
  Constant/1 -> Switch1/1
  Gain/1 -> Switch1/3
  Switch1/1 -> force/1
  Switch/1 -> Gain/1
  Gain2/1 -> Switch/3
  Gain4/1 -> Switch/1
  Sum/1 -> Gain4/1
  Gain3/1 -> Sum1/1, Sum/1
  pos/1 -> Switch1/2, Gain3/1
  Gain1/1 -> Sum/2
  Math Function/1 -> Gain5/1, Gain1/1
  vel/1 -> Math Function/1, Switch/2

== system water_hopper_biped_FCPG_split/leg R/Subsystem ==
  pos : Inport
  vel : Inport  Port=2
  Constant : Constant  Value=0
  Gain : Gain  Gain=C_d*density
  Gain1 : Gain  Gain=-0.5
  Gain2 : Gain  Gain=S1
  Gain3 : Gain  Gain=g
  Gain4 : Gain  Gain=S2
  Gain5 : Gain  Gain=0.5
  Math Function : Math  Operator=square  SaturateOnIntegerOverflow=on
  Sum : Sum  Inputs=-+|
  Sum1 : Sum  Inputs=-+|
  Switch : Switch  ZeroCross=off
  Switch1 : Switch
  force : Outport
  wires:
  vel/1 -> Switch/2, Math Function/1
  Math Function/1 -> Gain1/1, Gain5/1
  Gain1/1 -> Sum/2
  pos/1 -> Gain3/1, Switch1/2
  Gain3/1 -> Sum/1, Sum1/1
  Sum/1 -> Gain4/1
  Gain4/1 -> Switch/1
  Gain2/1 -> Switch/3
  Switch/1 -> Gain/1
  Switch1/1 -> force/1
  Gain/1 -> Switch1/3
  Constant/1 -> Switch1/1
  Sum1/1 -> Gain2/1
  Gain5/1 -> Sum1/2

== system water_hopper_biped_FCPG_split/CPG_Network/Subsystem/enable ==
  in : Inport
  Constant1 : Constant
  Constant2 : Constant
  Derivative : Derivative
  Gain : Gain  Gain=.5
  Gain1 : Gain  Gain=.5
  Sign : Signum
  Sum1 : Sum  Inputs=|++
  Sum2 : Sum  Inputs=|-+
  pos : Outport
  neg : Outport  Port=2
  wires:
  Derivative/1 -> Sign/1
  Constant1/1 -> Sum1/2
  Sign/1 -> Sum2/1, Sum1/1
  Gain/1 -> pos/1
  in/1 -> Derivative/1
  Sum1/1 -> Gain/1
  Constant2/1 -> Sum2/2
  Gain1/1 -> neg/1
  Sum2/1 -> Gain1/1

== system water_hopper_biped_FCPG_split/CPG_Network/Subsystem1/enable ==
  in : Inport
  Constant1 : Constant
  Constant2 : Constant
  Derivative : Derivative
  Gain : Gain  Gain=.5
  Gain1 : Gain  Gain=.5
  Sign : Signum
  Sum1 : Sum  Inputs=|++
  Sum2 : Sum  Inputs=|-+
  pos : Outport
  neg : Outport  Port=2
  wires:
  Derivative/1 -> Sign/1
  Constant1/1 -> Sum1/2
  Sign/1 -> Sum2/1, Sum1/1
  Gain/1 -> pos/1
  in/1 -> Derivative/1
  Sum1/1 -> Gain/1
  Constant2/1 -> Sum2/2
  Gain1/1 -> neg/1
  Sum2/1 -> Gain1/1
